simulink model "mrsDiffDriveModel"  (R2018a)
settings: Solver=VariableStepAuto  StartTime=0.0  StopTime=inf  FixedStep=0.01  RelTol=1e-3  EnableMultiTasking=on
PreLoadFcn:
  | sampleTime = 0.05;
  | 
  | % Vehicle Parameters
  | R = 0.1;
  | L = 0.5;
values from neighbouring files (symbols this model uses):
  C1 = x    (= 500)    [Augmented_States.m]    (also in tesla1.m)
  C2 = y + r    (= 510)    [Augmented_States.m]    (also in tesla1.m)
  cBW = 1/bRef    (= 0.1)    [Augmented_States.m]    (also in tesla1.m)
  Waypoint = WaypointA(x,y,l,r)    [tesla1.m]
undefined symbols (not defined in the file or in its folder): magnitude
libraries: mobileRoboticsLib x2, cstblocks x1, dspsrcs4 x1
settings Model: EnablePacing=on  Creator=scastro  LastModifiedBy=shravan
settings DataIOCC: LimitDataPoints=on
settings OptimizationCC: LifeSpan=inf
settings DebuggingCC: AllowSymbolicDim=off  SFUnexpectedBacktrackingDiag=warning  SFNoUnconditionalDefaultTransitionDiag=warning  SFExecutionAtInitializationDiag=none
settings CodeAppCC: StateflowObjectComments=on
settings GRTTargetCC: TargetLangStandard=C89/C90 (ANSI)  GeneratePreprocessorConditionals=Disable all
settings ConfigComp: CovMetricSettings=dw  CovHtmlReporting=on  CovSaveCumulativeToWorkspaceVar=on  CovSaveSingleToWorkspaceVar=on  CovExternalEMLEnable=off  CovSFcnEnable=off
settings SimscapeCC: SimscapeNominalValues="[{\"value\":\"10\",\"unit\":\"V\"},{\"value\":\"1\",\"unit\":\"A\"},{\"value\":\"10\",\"unit\":\"N*m\"},{\"value\":\"10\",\"unit\":\"bar\"},{\"value\":\"100\",\"unit\":\"kJ/kg\"},{\"value\":\"1\",\"unit\":\"kW\"},{\"value\":\"300\",\"unit\":\"K\"},{\"value\":\"100\",\"unit\":\"cm^3/s\"},{\"value\":\"1\",\"unit\":\"kN\"},{\"value\":\"1\",\"unit\":\"g/cm^3\"},{\"value\":\"1\",\"unit\":\"l\"},{\"value\":\"1\",\"unit\":\"cm^2\"},{\"value\":\"60\",\"unit\":\"Hz\"}]"  SimscapeLogType=all  SimscapeLogDataHistory=10000
settings ConfigurationSet: Description=SimMechanics 2G
settings ExplorerConfigSet: InternalSimMechanicsExplorerSettings="<ExplorerConfiguration><canonicalview>default</canonicalview><AnimationSetting><BasePlaybackSpeed>1.0</BasePlaybackSpeed><PlaybackSpeedFactor>1.0</PlaybackSpeedFactor></AnimationSetting><TilePanel><TileInfo><Tiles Columns=\"1\" Count=\"1\" Rows=\"1\"><Column Weight=\"1\"/><Row Weight=\"1\"/><Tile Height=\"1\" Width=\"1\" X=\"0\" Y=\"0\"/></Tiles></TileInfo><SceneInfo><SceneViewer><BGColor><R>0.60000002384185791</R><G>0.60000002384185791</G><B>0.60000002384185791</B></BGColor><Camera><DoPerspective>off</DoPerspective><Position><X>-1.70656042355848525</X><Y>-0.974920623359631922</Y><Z>4.72930454537082046</Z></Position><Center><X>0.552860638431633689</X><Y>1.42025063411503494</Y><Z>1.4843509506914252</Z></Center><Up><X>0.664249622453917166</X><Y>0.300615402055903091</Y><Z>0.684399604848363485</Z></Up><ViewLimDist>1</ViewLimDist><YLim>2.77881717169207398</YLim><XLim>3.55928742670435394</XLim></Camera></SceneViewer></SceneInfo></TilePanel><MechEditorPanel><Cameras/><GfxPanelCameraMap/><VideoCreator><PlaybackSpeedRatio>1.0</PlaybackSpeedRatio><FrameRate>30</FrameRate><VideoFormat>Motion JPEG AVI</VideoFormat><FrameSize>auto</FrameSize></VideoCreator></MechEditorPanel></ExplorerConfiguration>"

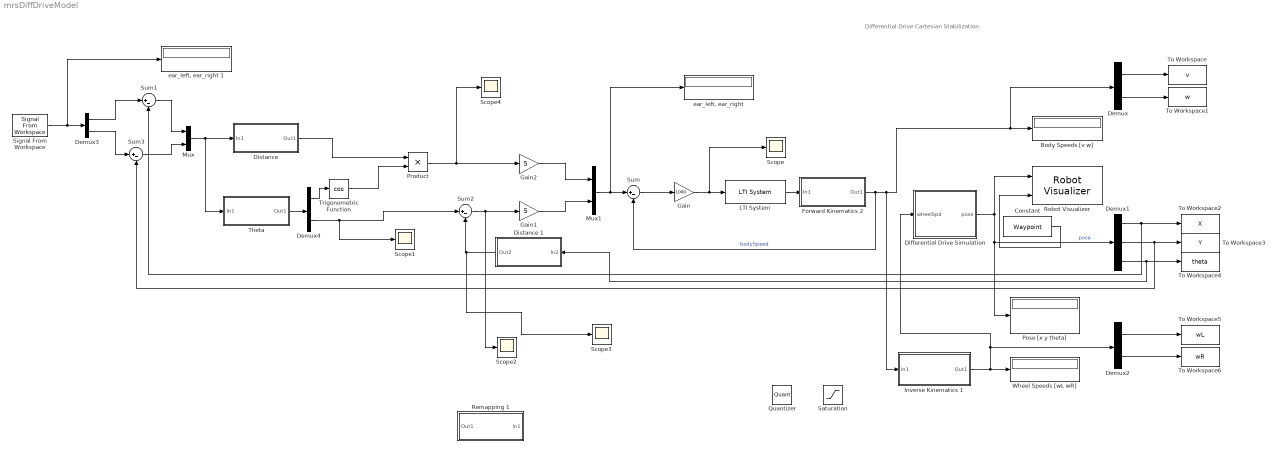
== system mrsDiffDriveModel ==
  note: Differential Drive Cartesian Stabilization
  Body Speeds [v w] : Display
  Constant : Constant  Value=Waypoint  SampleTime=sampleTime
  Demux{,2..4} (4 alike) : Demux  Outputs=2
  Demux1 : Demux  Outputs=3
  Differential Drive Simulation : Subsystem  AncestorBlock=mobileRoboticsLib/Kinematic Models/Differential Drive/Differential Drive Simulation  OverrideUsingVariant=mode==2  mask(Differential Drive Simulation){wheelRadius=R, wheelBase=L, initX=C1, initY=C2, initAngle=0, Ts=sampleTime}
      mask prompts: wheelRadius "Wheel Radius [m]"; wheelBase "Wheelbase [m]"; initX "Initial X Position [m]"; initY "Initial Y Position [m]"; initAngle "Initial Angle [rad]"; Ts "Sample Time"
      mask help:
      | Simulates the kinematics of a differential drive vehicle from a specified initial pose.
      |
      | Input: Left and right wheel speeds [wL; wR], in rad/s
      |
      | Output: Pose [x; y; theta], in m, m, and rad
      |
      | Set the Sample Time parameter to 0 for continuous-time simulation, or a positive number for discrete-time simulation.
      mask Help: web('matlab:edit mrsDocDifferentialDrive')
      mask Callback Ts:
      | Ts = evalin('base',get_param(gcb,'Ts'));
      | blk = [gcb '/Generic Robot Simulation/Velocity Integrator'];
      | if Ts > 0
      |     set_param(blk,'OverrideUsingVariant','mode==2');
      | else
      |     set_param(blk,'OverrideUsingVariant','mode==1');
      | end
  "Distance " : Subsystem
  Distance 1 : Subsystem
  Forward Kinematics 2 : Subsystem
  Gain : Gain  Gain=1000
  Gain1 : Gain  Gain=5
  Gain2 : Gain  Gain=5
  Inverse Kinematics 1 : Subsystem
  LTI System : cstblocks/LTI System  sys=Plant  IC=[0 0 0 0]
  Mux : Mux  Inputs=2
  Mux1 : Mux  Inputs=2
  Pose [x y theta] : Display
  Product : Product
  Quantizer : Quantizer
  Remapping 1 : Subsystem
  Robot Visualizer : mobileRoboticsLib/Environments/Robot Visualizer  Priority=99  robotRadius=0.1  showTrajectory=on  hasWaypoints=on  hasLidar=off  sensorOffset=[ 0 0 ]  scanAngles=scanAngles  hasObjDetector=off  objDetectorOffset=[ 0, 0 ]  objDetectorAngle=0  objDetectorFOV=pi/4  objDetectorMaxRange=5  objectColors=[ 1, 0, 0; 0, 1, 0; 0, 0, 1 ]  objectMarkers='s'
      settings: SourceProductName=Mobile Robotics Simulation Library
  Saturation : Saturate
  Scope{,1..4} (5 alike) : Scope
  Signal From Workspace : dspsrcs4/Signal From Workspace  X=Cartesian  Ts=cBW  nsamps=1  OutputAfterFinalValue=Holding final value  ignoreOrWarnInputAndFrameLengths=off  OutputFrames=off
  Sum{,1..3} (4 alike) : Sum  Inputs=|+-
  "Theta " : Subsystem
  To Workspace : ToWorkspace  VariableName=v  SampleTime=-1
  To Workspace1 : ToWorkspace  VariableName=w  SampleTime=-1
  To Workspace2 : ToWorkspace  VariableName=X  SampleTime=sampleTime
  To Workspace3 : ToWorkspace  VariableName=Y  SampleTime=-1
  To Workspace4 : ToWorkspace  VariableName=theta  SampleTime=-1
  To Workspace5 : ToWorkspace  VariableName=wL  SampleTime=-1
  To Workspace6 : ToWorkspace  VariableName=wR  SampleTime=-1
  Trigonometric Function : Trigonometry  Operator=cos
  Wheel Speeds [wL wR] : Display
  "ear_left, ear_right " : Display
  "ear_left, ear_right 1" : Display
  wires:
  Differential Drive Simulation/1(pose) -> Demux1/1, Pose [x y theta]/1, Robot Visualizer/1  "pose"
  Forward Kinematics 2/1(Out1) -> Sum/2, Inverse Kinematics 1/1(In1), Demux/1, Body Speeds [v w]/1  "bodySpeed"
  Demux/1 -> To Workspace/1
  Demux/2 -> To Workspace1/1
  Demux1/1 -> Sum1/2, To Workspace2/1
  Demux1/2 -> Sum3/2, To Workspace3/1
  Demux2/1 -> To Workspace5/1
  Demux2/2 -> To Workspace6/1
  Gain2/1 -> Mux1/1
  Gain/1 -> LTI System/1, Scope/1
  Sum/1 -> Gain/1
  Constant/1 -> Robot Visualizer/2
  LTI System/1 -> Forward Kinematics 2/1(In1)
  Inverse Kinematics 1/1(Out1) -> Demux2/1, Differential Drive Simulation/1(wheelSpd), Wheel Speeds [wL wR]/1
  Gain1/1 -> Mux1/2
  Demux1/3 -> Distance 1/1(In2), To Workspace4/1
  "Distance "/1(Out1) -> Product/1
  Trigonometric Function/1 -> Product/2
  Product/1 -> Scope4/1, Gain2/1
  Mux1/1 -> "ear_left, ear_right "/1, Sum/1
  Sum2/1 -> Scope2/1, Gain1/1
  Signal From Workspace/1 -> "ear_left, ear_right 1"/1, Demux3/1
  Demux3/1 -> Sum1/1
  Demux3/2 -> Sum3/1
  Sum3/1 -> Mux/2
  Sum1/1 -> Mux/1
  Mux/1 -> "Theta "/1(In1), "Distance "/1(In1)
  Distance 1/1(Out2) -> Scope3/1, Sum2/2
  Demux4/1 -> Trigonometric Function/1
  Demux4/2 -> Scope1/1, Sum2/1
  "Theta "/1(Out1) -> Demux4/1

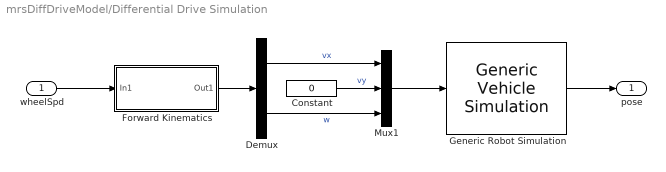
== system mrsDiffDriveModel/Differential Drive Simulation ==
  wheelSpd : Inport
  Constant : Constant  Value=0
  Demux : Demux  Outputs=2
  "Forward Kinematics " : Subsystem
  Generic Robot Simulation : mobileRoboticsLib/Utilities/Generic Vehicle Simulation  initX=initX  initY=initY  initAngle=initAngle  Ts=Ts
      link override Velocity Integrator: OverrideUsingVariant=mode==2
      settings: SourceProductName=Mobile Robotics Simulation Toolbox
  Mux1 : Mux  Inputs=3
  pose : Outport
  wires:
  Generic Robot Simulation/1 -> pose/1
  "Forward Kinematics "/1(Out1) -> Demux/1
  wheelSpd/1 -> "Forward Kinematics "/1(In1)
  Constant/1 -> Mux1/2  "vy"
  Demux/2 -> Mux1/3  "w"
  Demux/1 -> Mux1/1  "vx"
  Mux1/1 -> Generic Robot Simulation/1

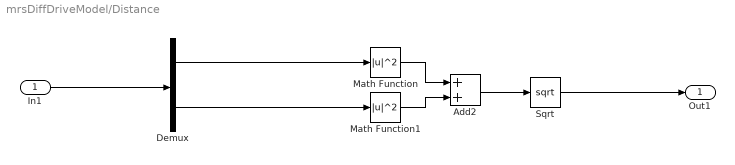
== system mrsDiffDriveModel/Distance  ==
  In1 : Inport
  Add2 : Sum
  Demux : Demux  Outputs=2
  Math Function : Math  Operator=magnitude^2  SaturateOnIntegerOverflow=on
  Math Function1 : Math  Operator=magnitude^2  SaturateOnIntegerOverflow=on
  Sqrt : Sqrt  SaturateOnIntegerOverflow=on
  Out1 : Outport
  wires:
  In1/1 -> Demux/1
  Demux/1 -> Math Function/1
  Demux/2 -> Math Function1/1
  Math Function/1 -> Add2/1
  Math Function1/1 -> Add2/2
  Add2/1 -> Sqrt/1
  Sqrt/1 -> Out1/1

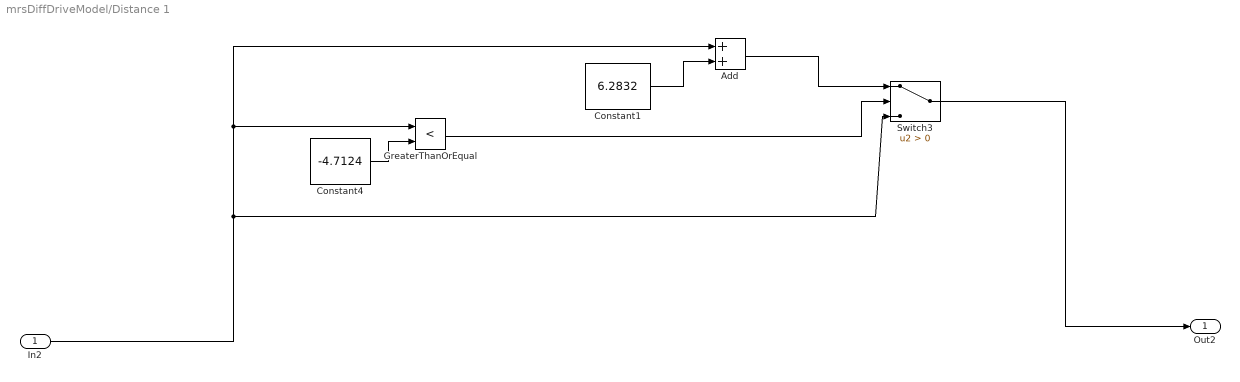
== system mrsDiffDriveModel/Distance 1 ==
  In2 : Inport
  Add : Sum
  Constant1 : Constant  Value=6.2832
  Constant4 : Constant  Value=-4.7124
  GreaterThanOrEqual : RelationalOperator  Operator=<  OutDataTypeStr=boolean  RndMeth=Simplest
  Switch3 : Switch  Criteria=u2 > Threshold
  Out2 : Outport
  wires:
  Switch3/1 -> Out2/1
  Constant4/1 -> GreaterThanOrEqual/2
  GreaterThanOrEqual/1 -> Switch3/2
  In2/1 -> Switch3/3, Add/1, GreaterThanOrEqual/1
  Constant1/1 -> Add/2
  Add/1 -> Switch3/1

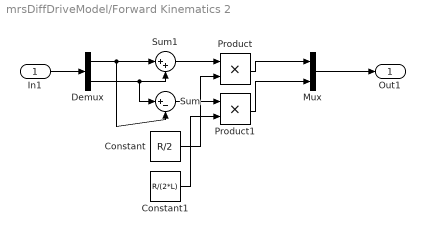
== system mrsDiffDriveModel/Forward Kinematics 2 ==
  In1 : Inport
  Constant : Constant  Value=R/2
  Constant1 : Constant  Value=R/(2*L)
  Demux : Demux  Outputs=2
  Mux : Mux  Inputs=2
  Product : Product
  Product1 : Product
  Sum : Sum  Inputs=|+-
  Sum1 : Sum  Inputs=|++
  Out1 : Outport
  wires:
  In1/1 -> Demux/1
  Product1/1 -> Mux/2
  Mux/1 -> Out1/1
  Product/1 -> Mux/1
  Demux/1 -> Sum/2, Sum1/1
  Demux/2 -> Sum/1, Sum1/2
  Sum1/1 -> Product/1
  Constant/1 -> Product/2
  Sum/1 -> Product1/1
  Constant1/1 -> Product1/2

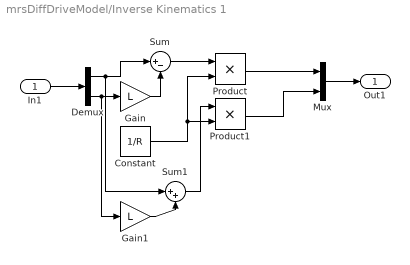
== system mrsDiffDriveModel/Inverse Kinematics 1 ==
  In1 : Inport
  Constant : Constant  Value=1/R
  Demux : Demux  Outputs=2
  Gain : Gain  Gain=L
  Gain1 : Gain  Gain=L
  Mux : Mux  Inputs=2
  Product : Product
  Product1 : Product
  Sum : Sum  Inputs=|+-
  Sum1 : Sum  Inputs=|++
  Out1 : Outport
  wires:
  Mux/1 -> Out1/1
  In1/1 -> Demux/1
  Demux/2 -> Gain1/1, Gain/1
  Demux/1 -> Sum1/1, Sum/1
  Gain/1 -> Sum/2
  Sum/1 -> Product/1
  Constant/1 -> Product1/2, Product/2
  Sum1/1 -> Product1/1
  Product/1 -> Mux/1
  Product1/1 -> Mux/2
  Gain1/1 -> Sum1/2

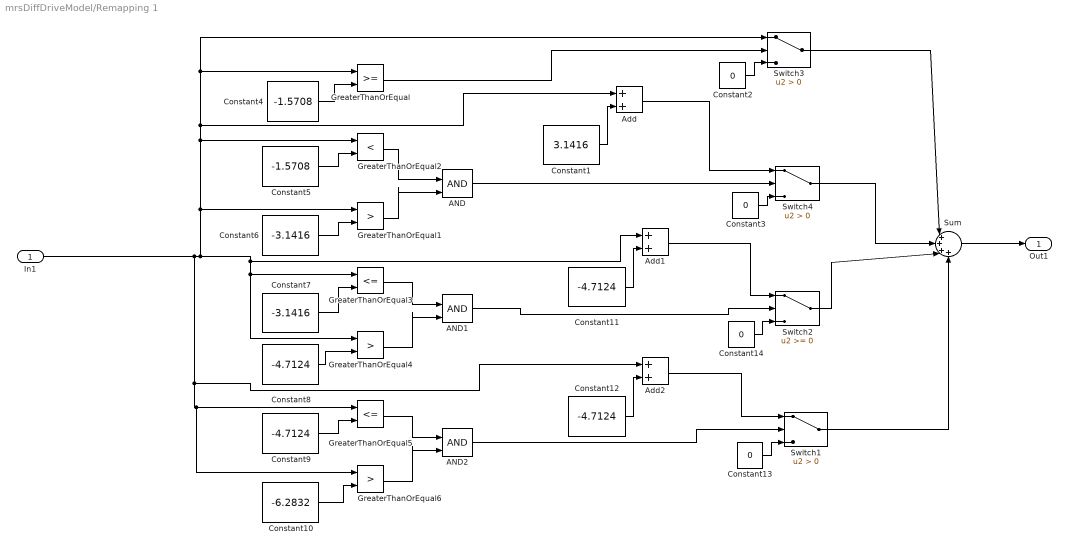
== system mrsDiffDriveModel/Remapping 1 ==
  In1 : Inport
  AND : Logic  IconShape=distinctive  AllPortsSameDT=off  OutDataTypeStr=boolean
  AND1 : Logic  IconShape=distinctive  AllPortsSameDT=off  OutDataTypeStr=boolean
  AND2 : Logic  IconShape=distinctive  AllPortsSameDT=off  OutDataTypeStr=boolean
  Add : Sum
  Add1 : Sum
  Add2 : Sum
  Constant1 : Constant  Value=3.1416
  Constant10 : Constant  Value=-6.2832
  Constant{8..9,11..12} (4 alike) : Constant  Value=-4.7124
  Constant{2..3,13..14} (4 alike) : Constant  Value=0
  Constant4 : Constant  Value=-1.5708
  Constant5 : Constant  Value=-1.5708
  Constant6 : Constant  Value=-3.1416
  Constant7 : Constant  Value=-3.1416
  GreaterThanOrEqual : RelationalOperator  OutDataTypeStr=boolean  RndMeth=Simplest
  GreaterThanOrEqual1 : RelationalOperator  Operator=>  OutDataTypeStr=boolean  RndMeth=Simplest
  GreaterThanOrEqual2 : RelationalOperator  Operator=<  OutDataTypeStr=boolean  RndMeth=Simplest
  GreaterThanOrEqual3 : RelationalOperator  Operator=<=  OutDataTypeStr=boolean  RndMeth=Simplest
  GreaterThanOrEqual4 : RelationalOperator  Operator=>  OutDataTypeStr=boolean  RndMeth=Simplest
  GreaterThanOrEqual5 : RelationalOperator  Operator=<=  OutDataTypeStr=boolean  RndMeth=Simplest
  GreaterThanOrEqual6 : RelationalOperator  Operator=>  OutDataTypeStr=boolean  RndMeth=Simplest
  Sum : Sum  Inputs=|++++
  Switch1 : Switch  Criteria=u2 > Threshold
  Switch2 : Switch
  Switch3 : Switch  Criteria=u2 > Threshold
  Switch4 : Switch  Criteria=u2 > Threshold
  Out1 : Outport
  wires:
  Constant2/1 -> Switch3/3
  Constant3/1 -> Switch4/3
  Constant4/1 -> GreaterThanOrEqual/2
  Constant5/1 -> GreaterThanOrEqual2/2
  Constant6/1 -> GreaterThanOrEqual1/2
  Constant7/1 -> GreaterThanOrEqual3/2
  Constant8/1 -> GreaterThanOrEqual4/2
  Constant9/1 -> GreaterThanOrEqual5/2
  Constant10/1 -> GreaterThanOrEqual6/2
  GreaterThanOrEqual2/1 -> AND/1
  GreaterThanOrEqual1/1 -> AND/2
  GreaterThanOrEqual3/1 -> AND1/1
  GreaterThanOrEqual4/1 -> AND1/2
  GreaterThanOrEqual5/1 -> AND2/1
  GreaterThanOrEqual6/1 -> AND2/2
  In1/1 -> Add2/1, GreaterThanOrEqual6/1, GreaterThanOrEqual5/1, Add1/1, GreaterThanOrEqual4/1, GreaterThanOrEqual3/1, GreaterThanOrEqual1/1, GreaterThanOrEqual2/1, Add/1, Switch3/1, GreaterThanOrEqual/1
  Constant12/1 -> Add2/2
  Constant1/1 -> Add/2
  Constant11/1 -> Add1/2
  GreaterThanOrEqual/1 -> Switch3/2
  Constant13/1 -> Switch1/3
  Constant14/1 -> Switch2/3
  AND/1 -> Switch4/2
  AND1/1 -> Switch2/2
  Add/1 -> Switch4/1
  Add1/1 -> Switch2/1
  Add2/1 -> Switch1/1
  AND2/1 -> Switch1/2
  Switch3/1 -> Sum/1
  Switch4/1 -> Sum/2
  Switch2/1 -> Sum/3
  Switch1/1 -> Sum/4
  Sum/1 -> Out1/1

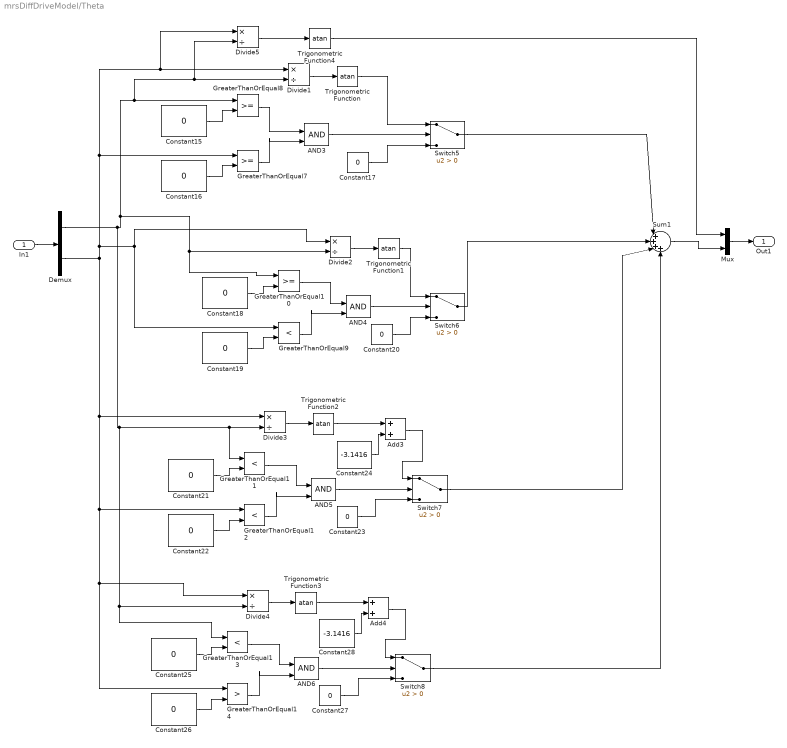
== system mrsDiffDriveModel/Theta  ==
  In1 : Inport
  AND{3..6} (4 alike) : Logic  IconShape=distinctive  AllPortsSameDT=off  OutDataTypeStr=boolean
  Add3 : Sum
  Add4 : Sum
  Constant{15..23,25..27} (12 alike) : Constant  Value=0
  Constant24 : Constant  Value=-3.1416
  Constant28 : Constant  Value=-3.1416
  Demux : Demux  Outputs=2
  Divide{1..5} (5 alike) : Product  Inputs=*/
  GreaterThanOrEqual10 : RelationalOperator  OutDataTypeStr=boolean  RndMeth=Simplest
  GreaterThanOrEqual{9,11..13} (4 alike) : RelationalOperator  Operator=<  OutDataTypeStr=boolean  RndMeth=Simplest
  GreaterThanOrEqual14 : RelationalOperator  Operator=>  OutDataTypeStr=boolean  RndMeth=Simplest
  GreaterThanOrEqual7 : RelationalOperator  OutDataTypeStr=boolean  RndMeth=Simplest
  GreaterThanOrEqual8 : RelationalOperator  OutDataTypeStr=boolean  RndMeth=Simplest
  Mux : Mux  Inputs=2
  Sum1 : Sum  Inputs=|++++
  Switch{5..8} (4 alike) : Switch  Criteria=u2 > Threshold
  Trigonometric Function{,1..4} (5 alike) : Trigonometry  Operator=atan
  Out1 : Outport
  wires:
  In1/1 -> Demux/1
  Divide1/1 -> Trigonometric Function/1
  Constant16/1 -> GreaterThanOrEqual7/2
  GreaterThanOrEqual7/1 -> AND3/2
  Constant15/1 -> GreaterThanOrEqual8/2
  Demux/1 -> Divide4/2, GreaterThanOrEqual13/1, GreaterThanOrEqual11/1, Divide3/2, Divide2/2, GreaterThanOrEqual10/1, Divide5/2, Divide1/2, GreaterThanOrEqual8/1
  GreaterThanOrEqual8/1 -> AND3/1
  Constant17/1 -> Switch5/3
  AND3/1 -> Switch5/2
  Demux/2 -> Divide4/1, GreaterThanOrEqual14/1, GreaterThanOrEqual12/1, Divide3/1, GreaterThanOrEqual9/1, Divide2/1, Divide5/1, Divide1/1, GreaterThanOrEqual7/1
  Trigonometric Function/1 -> Switch5/1
  Trigonometric Function1/1 -> Switch6/1
  AND4/1 -> Switch6/2
  GreaterThanOrEqual10/1 -> AND4/1
  Constant19/1 -> GreaterThanOrEqual9/2
  Constant20/1 -> Switch6/3
  GreaterThanOrEqual9/1 -> AND4/2
  Constant18/1 -> GreaterThanOrEqual10/2
  Divide2/1 -> Trigonometric Function1/1
  AND5/1 -> Switch7/2
  GreaterThanOrEqual11/1 -> AND5/1
  Divide3/1 -> Trigonometric Function2/1
  GreaterThanOrEqual12/1 -> AND5/2
  Constant22/1 -> GreaterThanOrEqual12/2
  Constant21/1 -> GreaterThanOrEqual11/2
  Constant23/1 -> Switch7/3
  Trigonometric Function2/1 -> Add3/1
  Constant24/1 -> Add3/2
  Add3/1 -> Switch7/1
  Constant26/1 -> GreaterThanOrEqual14/2
  GreaterThanOrEqual14/1 -> AND6/2
  Constant28/1 -> Add4/2
  Constant27/1 -> Switch8/3
  AND6/1 -> Switch8/2
  Add4/1 -> Switch8/1
  Divide4/1 -> Trigonometric Function3/1
  GreaterThanOrEqual13/1 -> AND6/1
  Constant25/1 -> GreaterThanOrEqual13/2
  Trigonometric Function3/1 -> Add4/1
  Switch5/1 -> Sum1/1
  Switch6/1 -> Sum1/2
  Switch7/1 -> Sum1/3
  Switch8/1 -> Sum1/4
  Sum1/1 -> Mux/2
  Divide5/1 -> Trigonometric Function4/1
  Trigonometric Function4/1 -> Mux/1
  Mux/1 -> Out1/1

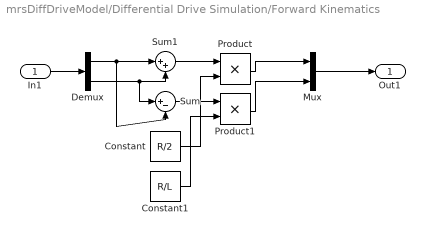
== system mrsDiffDriveModel/Differential Drive Simulation/Forward Kinematics  ==
  In1 : Inport
  Constant : Constant  Value=R/2
  Constant1 : Constant  Value=R/L
  Demux : Demux  Outputs=2
  Mux : Mux  Inputs=2
  Product : Product
  Product1 : Product
  Sum : Sum  Inputs=|+-
  Sum1 : Sum  Inputs=|++
  Out1 : Outport
  wires:
  In1/1 -> Demux/1
  Product1/1 -> Mux/2
  Mux/1 -> Out1/1
  Product/1 -> Mux/1
  Demux/1 -> Sum/2, Sum1/1
  Demux/2 -> Sum/1, Sum1/2
  Sum1/1 -> Product/1
  Constant/1 -> Product/2
  Sum/1 -> Product1/1
  Constant1/1 -> Product1/2
